simulink model "Control_Block_r1"  (R2020a)
settings: Solver=VariableStepAuto  StartTime=0.0  StopTime=10.0  RelTol=1e-3
undefined symbols (not defined in the file): sigbuilder_block
libraries: fuzblock x1
settings Model: Creator=chris  LastModifiedBy=chris

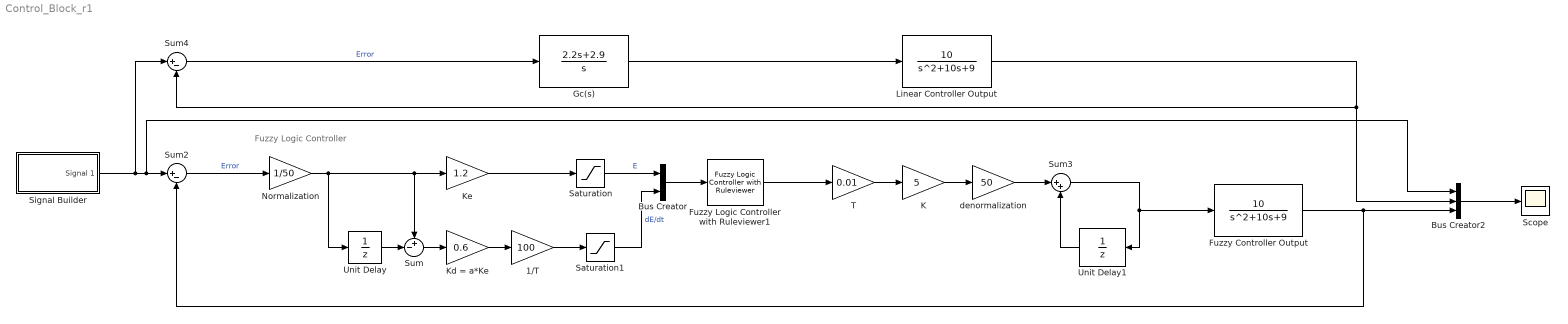
== system Control_Block_r1 ==
  note: Fuzzy Logic Controller
  1/T : Gain  Gain=100
  Bus Creator : BusCreator  Inputs=2
  Bus Creator2 : BusCreator  Inputs=3
  Fuzzy Controller Output : TransferFcn  Numerator=[10]  Denominator=[1 10 9]
  Fuzzy Logic Controller with Ruleviewer1 : fuzblock/Fuzzy Logic  Controller  with Ruleviewer  fismatrix=FLC  Ts=0.01
  Gc(s) : TransferFcn  Numerator=[0 2.2 2.9]  Denominator=[1 0]
  K : Gain  Gain=5
  Kd = a*Ke : Gain  Gain=0.6
  Ke : Gain  Gain=1.2
  Linear Controller Output : TransferFcn  Numerator=[10]  Denominator=[1 10 9]
  Normalization : Gain  Gain=1/50
  Saturation : Saturate  UpperLimit=1  LowerLimit=-1
  Saturation1 : Saturate  UpperLimit=1  LowerLimit=-1
  Scope : Scope
  Signal Builder : Subsystem  Tag=STV Subsys  LoadFcn=sigbuilder_block('load',[437.6 199.2 550.4 400 ]);  StartFcn=sigbuilder_block('start');  StopFcn=sigbuilder_block('stop');  ClipboardFcn=sigbuilder_block('clipboard');  mask(Sigbuilder block){tuvar=[0:10]}
      mask help: Simulink:masks:SigbuilderBlock_MD
      mask init:
      | if ~strcmp(get_param(bdroot(gcbh),'SimulationStatus'),'stopped') tuvar = sigbuilder_block('maskInit'); end
      settings: CopyFcn=sigbuilder_block('copy');  DeleteFcn=sigbuilder_block('delete');  ModelCloseFcn=sigbuilder_block('modelClose');  PreSaveFcn=sigbuilder_block('preSave');  PauseFcn=sigbuilder_block('pause');  ContinueFcn=sigbuilder_block('continue');  NameChangeFcn=sigbuilder_block('namechange');  OpenFcn=sigbuilder_block('open',[437.6 199.2 550.4 400 ]);  CloseFcn=sigbuilder_block('close');
      mask Display: plot(0, 0, 100, 100,[2, 2, 32, 32, 2], [68, 8, 8, 68, 68],[32, 2], [38, 38], [32, 19, 2],[53, 60, 44], [32, 17, 17, 2],[16, 16, 31, 31]);txt = getActiveGroup(gcbh);text(2, 100, txt,'verticalAlignment', 'top');
  Sum : Sum  Inputs=+-|
  Sum2 : Sum  Inputs=|+-
  Sum3 : Sum  Inputs=|++
  Sum4 : Sum  Inputs=|+-
  T : Gain  Gain=0.01
  Unit Delay : UnitDelay  SampleTime=-1  HasFrameUpgradeWarning=on
  Unit Delay1 : UnitDelay  SampleTime=-1  HasFrameUpgradeWarning=on
  denormalization : Gain  Gain=50
  wires:
  Bus Creator2/1 -> Scope/1
  Sum4/1 -> Gc(s)/1  "Error"
  Gc(s)/1 -> Linear Controller Output/1
  Linear Controller Output/1 -> Sum4/2, Bus Creator2/2
  Bus Creator/1 -> Fuzzy Logic Controller with Ruleviewer1/1
  Fuzzy Logic Controller with Ruleviewer1/1 -> T/1
  Normalization/1 -> Ke/1, Sum/1, Unit Delay/1
  Ke/1 -> Saturation/1
  T/1 -> K/1
  Saturation1/1 -> Bus Creator/2  "dE/dt"
  Kd = a*Ke/1 -> 1/T/1
  denormalization/1 -> Sum3/1
  Unit Delay/1 -> Sum/2
  Sum/1 -> Kd = a*Ke/1
  Saturation/1 -> Bus Creator/1  "E"
  Unit Delay1/1 -> Sum3/2
  K/1 -> denormalization/1
  1/T/1 -> Saturation1/1
  Sum2/1 -> Normalization/1  "Error"
  Fuzzy Controller Output/1 -> Sum2/2, Bus Creator2/3
  Sum3/1 -> Fuzzy Controller Output/1, Unit Delay1/1
  Signal Builder/1(Signal 1) -> Sum2/1, Bus Creator2/1, Sum4/1

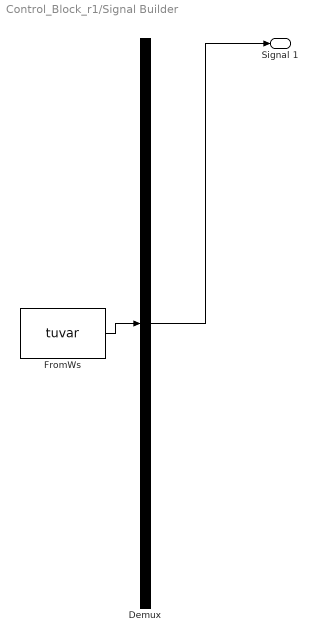
== system Control_Block_r1/Signal Builder ==
  Demux : Demux  Tag=STV Demux  Outputs=1
      settings: DisplayOption=none
  FromWs : FromWorkspace  Tag=STV FromWs  VariableName=tuvar
      SigBuilderData=|
      | common.afterFinalStr = 'Extrapolate'
      | common.sampleTime = 0
      | dataSet.timeRange = [0 10]
      | dataSet.name = 'Group 1'
      | sbobj.Groups.Name = 'Group 1'
      | sbobj.Groups.Signals.Name = 'Signal 1'
      | sbobj.Groups.Signals.XData = [0 4 4 8 8 10]
      | sbobj.Groups.Signals.YData = [60 60 20 20 40 40]
  Signal 1 : Outport  Tag=STV Outport
  wires:
  Demux/1 -> Signal 1/1
  FromWs/1 -> Demux/1
